simulink model "Wrapper_oClientServer_Model"  (R2024b)
settings: Solver=FixedStepDiscrete  StartTime=0.0  StopTime=10.0  FixedStep=0.05  RelTol=1e-3
undefined symbols (not defined in the file or in its folder): call_ServerService_getDataC, call_ServerService_setDataA, call_ServerService_setDataB, DataA, DataB, sut_ServerService_setDataA, sut_ServerService_setDataB, sut_step
settings Model: Tag=EP_AA_WRAPPER_TOPLEVEL  DataDictionary=Wrapper_oClientServer_Model.sldd  Creator=nabilekhoury  LastModifiedBy=nabilekhoury
settings OptimizationCC: DefaultParameterBehavior=Inlined  OptimizeBlockIOStorage=off  BufferReuse=off  ReuseModelBlockBuffer=off  GlobalBufferReuse=off  ExpressionFolding=off  EnableMemcpy=off  PassReuseOutputArgsAs=Individual arguments  LocalBlockOutputs=off  ZeroExternalMemoryAtStartup=off  ZeroInternalMemoryAtStartup=off  OptimizeDataStoreBuffers=off  BusAssignmentInplaceUpdate=off  OptimizationLevel=level0  OptimizationCustomize=off  EfficientTunableParamExpr=on
settings DebuggingCC: ParameterTunabilityLossMsg=error
settings ModelReferenceCC: ModelReferenceNumInstancesAllowed=Single
settings SFSimCC: MATLABDynamicMemAlloc=off  SimTargetLang=C++
settings RTWCC: Description=Embedded Coder  SystemTargetFile=ert.tlc  GenCodeOnly=on  TemplateMakefile=ert_default_tmf  CustomSourceCode="#include \"oClientServer_Model_adapter.h\""  CustomInitializer=sut_initialize();  TargetLang=C++
settings CodeAppCC: ForceParamTrailComments=on  IgnoreCustomStorageClasses=off  MaxIdLength=256  OperatorAnnotations=on  SimulinkDataObjDesc=on  SFDataObjDesc=on  CustomSymbolStrGlobalVar=w_$R$N$M  CustomSymbolStrType=w_$N$R$M_T  InsertBlockDesc=on
settings ERTTargetCC: TargetLangStandard=C++17 (ISO)  GenerateSampleERTMain=on  SupportAbsoluteTime=off  SupportNonFinite=off  SupportComplex=off  RootIOFormat=Structure reference  ERTCustomFileTemplate=example_file_process.tlc

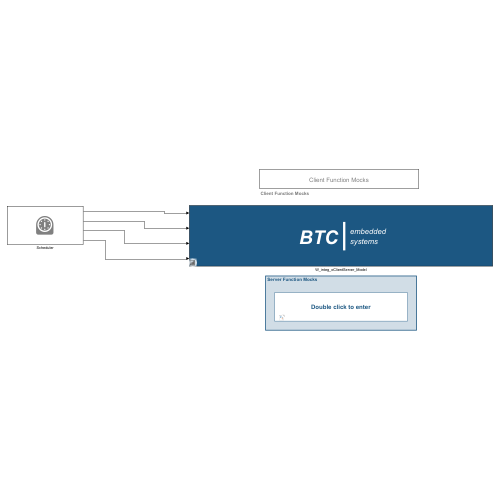
[thumbnail: Simulink's stored preview of the top-level diagram]
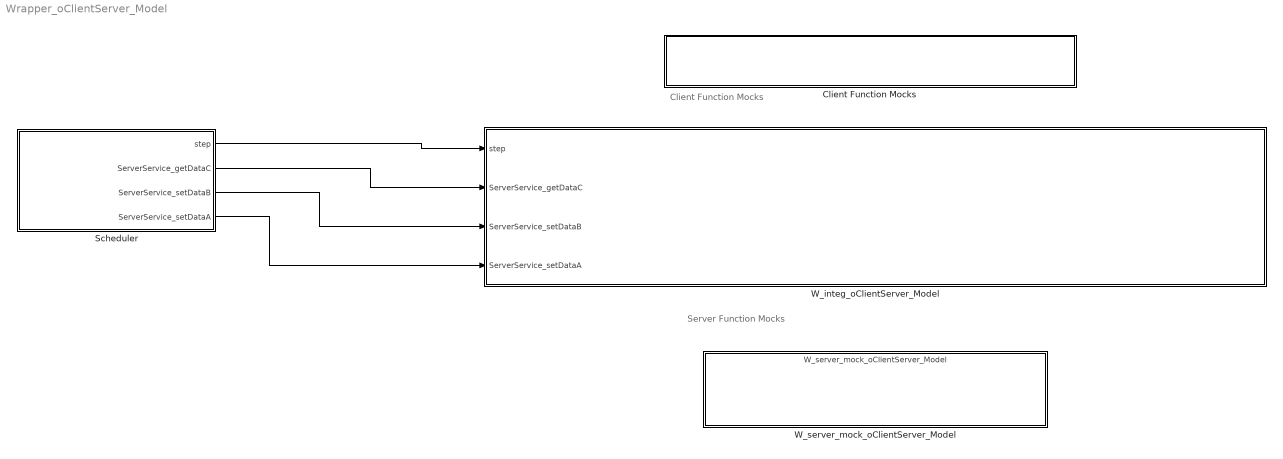
== system Wrapper_oClientServer_Model ==
  note: Client Function Mocks
  note: Server Function Mocks
  Client Function Mocks : Subsystem
      mask Display: color('gray'); disp('{\fontsize{16}Client Function Mocks}', 'texmode', 'on');
  Scheduler : Subsystem
      mask Display: disp('\color{gray}\fontsize{50}⏲', 'texmode', 'on');
  W_integ_oClientServer_Model : Subsystem  Variant=on  VariantControlMode=label  LabelModeActiveChoice=orig  PropagateVariantConditions=on
      settings: OpenFcn=open_system(gcb, 'mask');
      mask DialogControl DescGroupVar Prompt: BTC Embedded Systems SUT block
      mask DialogControl DescTextVar Prompt: This is the BTC Embedded Systems SUT block, referencing the original Adaptive AUTOSAR model.
      mask DialogControl DescButVar Prompt: Open original model...
      mask DialogControl DescButVar Callback: open_system('oClientServer_Model');
      mask Display: disp('\color{white}\it\fontsize{20}                          embedded\newline                          systems', 'texmode', 'on');disp('{{\color{white}\bf\fontsize{50}\it   BTC}  \fontsize{80}|      \color{black}\fontsize{20}\newline }', 'texmode','on');
  W_server_mock_oClientServer_Model : ModelReference  ModelNameDialog=W_server_mock_oClientServer_Model  SimulationMode=Normal  ScheduleRates=on  ModelReferenceVersion=1.1
      mask Display: disp('{\bf\fontsize{16}Double click to enter}', 'texmode', 'on');
  wires:
  Scheduler/2(ServerService_getDataC) -> W_integ_oClientServer_Model/2(ServerService_getDataC)
  Scheduler/4(ServerService_setDataA) -> W_integ_oClientServer_Model/4(ServerService_setDataA)
  Scheduler/3(ServerService_setDataB) -> W_integ_oClientServer_Model/3(ServerService_setDataB)
  Scheduler/1(step) -> W_integ_oClientServer_Model/1(step)

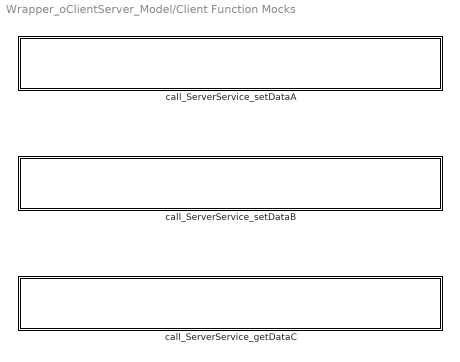
== system Wrapper_oClientServer_Model/Client Function Mocks ==
  call_ServerService_getDataC : Subsystem  TreatAsAtomicUnit=on
  call_ServerService_setDataA : Subsystem  TreatAsAtomicUnit=on
  call_ServerService_setDataB : Subsystem  TreatAsAtomicUnit=on

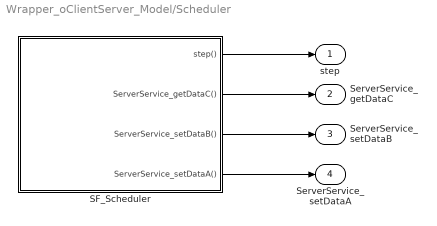
== system Wrapper_oClientServer_Model/Scheduler ==
  SF_Scheduler : Stateflow chart  TreatAsAtomicUnit=on
  step : Outport
  ServerService_getDataC : Outport  Port=2
  ServerService_setDataB : Outport  Port=3
  ServerService_setDataA : Outport  Port=4
  wires:
  SF_Scheduler/1(step()) -> step/1
  SF_Scheduler/2(ServerService_getDataC()) -> ServerService_getDataC/1
  SF_Scheduler/3(ServerService_setDataB()) -> ServerService_setDataB/1
  SF_Scheduler/4(ServerService_setDataA()) -> ServerService_setDataA/1

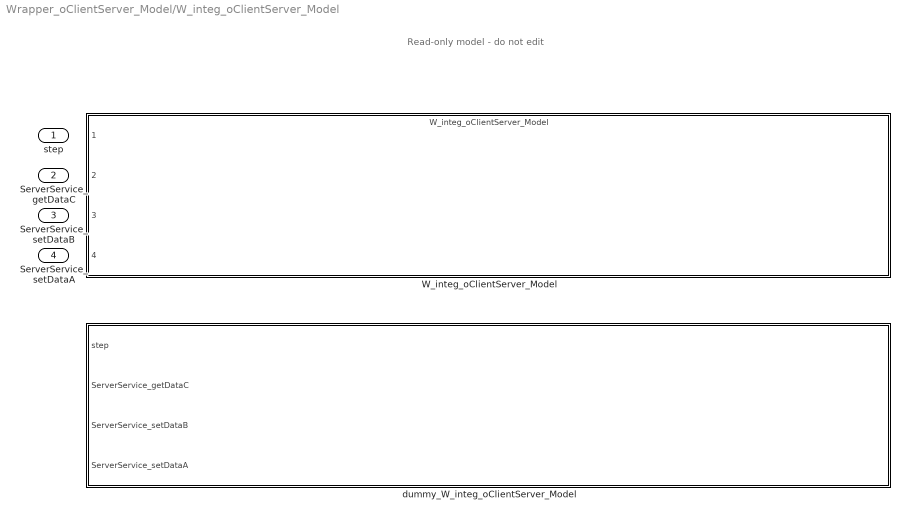
== system Wrapper_oClientServer_Model/W_integ_oClientServer_Model ==
  note: Read-only model - do not edit
  step : Inport
  ServerService_getDataC : Inport  Port=2
  ServerService_setDataB : Inport  Port=3
  ServerService_setDataA : Inport  Port=4
  W_integ_oClientServer_Model : ModelReference  Tag=BTC AUTOSAR Main Model Reference Block  ModelNameDialog=W_integ_oClientServer_Model  SimulationMode=Normal  ScheduleRates=on  VariantControl=orig  ModelReferenceVersion=1.2
  dummy_W_integ_oClientServer_Model : Subsystem  VariantControl=dummy

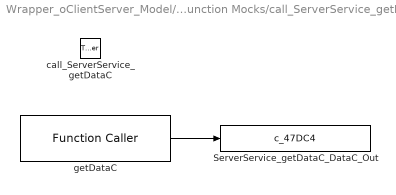
== system Wrapper_oClientServer_Model/Client Function Mocks/call_ServerService_getDataC ==
  call_ServerService_getDataC : TriggerPort  TriggerType=function-call  IsSimulinkFunction=on  FunctionName=call_ServerService_getDataC  VariantControl=(inherit)
  ServerService_getDataC_DataC_Out : DataStoreWrite  DataStoreName=c_47DC4  IndexOptions=Index vector (dialog)  Indices=1  OutputSizes=1
  getDataC : FunctionCaller  FunctionPrototype=DataC = sut_ServerService_getDataC()  OutputArgumentSpecifications=double(0)
  wires:
  getDataC/1 -> ServerService_getDataC_DataC_Out/1

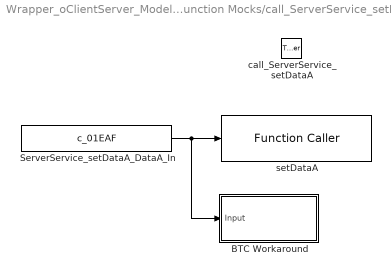
== system Wrapper_oClientServer_Model/Client Function Mocks/call_ServerService_setDataA ==
  call_ServerService_setDataA : TriggerPort  TriggerType=function-call  IsSimulinkFunction=on  FunctionName=call_ServerService_setDataA  VariantControl=(inherit)
  BTC Workaround : Subsystem
      settings: OpenFcn=open_system(gcb, 'mask');
      mask DialogControl DescGroupVar Prompt: BTC Embedded Systems MIL stabilizer
      mask DialogControl DescTextVar Prompt: The BTC Embedded Systems MIL stabilizer prevents a known Matlab 2023b issue that results in a crash. It has no effect on the signal. Do not edit its contents.
      mask Display: disp('\color[rgb]{0.11,0.34,0.51}\bf MIL stabilizer', 'texmode', 'on');
  ServerService_setDataA_DataA_In : DataStoreRead  DataStoreName=c_01EAF  IndexOptions=Index vector (dialog)  Indices=1  OutputSizes=1
  setDataA : FunctionCaller  FunctionPrototype=sut_ServerService_setDataA(DataA)  InputArgumentSpecifications=double(0)
  wires:
  ServerService_setDataA_DataA_In/1 -> setDataA/1, BTC Workaround/1(Input)

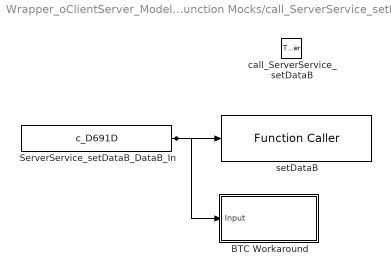
== system Wrapper_oClientServer_Model/Client Function Mocks/call_ServerService_setDataB ==
  call_ServerService_setDataB : TriggerPort  TriggerType=function-call  IsSimulinkFunction=on  FunctionName=call_ServerService_setDataB  VariantControl=(inherit)
  BTC Workaround : Subsystem
      settings: OpenFcn=open_system(gcb, 'mask');
      mask DialogControl DescGroupVar Prompt: BTC Embedded Systems MIL stabilizer
      mask DialogControl DescTextVar Prompt: The BTC Embedded Systems MIL stabilizer prevents a known Matlab 2023b issue that results in a crash. It has no effect on the signal. Do not edit its contents.
      mask Display: disp('\color[rgb]{0.11,0.34,0.51}\bf MIL stabilizer', 'texmode', 'on');
  ServerService_setDataB_DataB_In : DataStoreRead  DataStoreName=c_D691D  IndexOptions=Index vector (dialog)  Indices=1  OutputSizes=1
  setDataB : FunctionCaller  FunctionPrototype=sut_ServerService_setDataB(DataB)  InputArgumentSpecifications=double(0)
  wires:
  ServerService_setDataB_DataB_In/1 -> setDataB/1, BTC Workaround/1(Input)

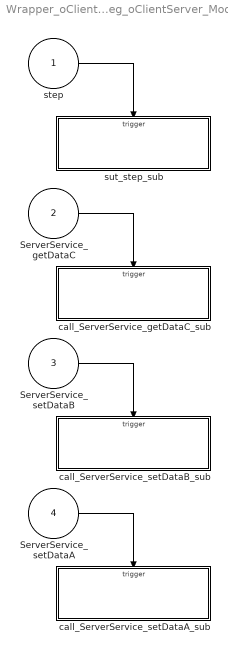
== system Wrapper_oClientServer_Model/W_integ_oClientServer_Model/dummy_W_integ_oClientServer_Model ==
  step : Inport  OutputFunctionCall=on
  ServerService_getDataC : Inport  Port=2  OutputFunctionCall=on
  ServerService_setDataB : Inport  Port=3  OutputFunctionCall=on
  ServerService_setDataA : Inport  Port=4  OutputFunctionCall=on
  call_ServerService_getDataC_sub : Subsystem  TreatAsAtomicUnit=on
  call_ServerService_setDataA_sub : Subsystem  TreatAsAtomicUnit=on
  call_ServerService_setDataB_sub : Subsystem  TreatAsAtomicUnit=on
  sut_step_sub : Subsystem  TreatAsAtomicUnit=on
  wires:
  step/1 -> sut_step_sub/Trigger
  ServerService_getDataC/1 -> call_ServerService_getDataC_sub/Trigger
  ServerService_setDataB/1 -> call_ServerService_setDataB_sub/Trigger
  ServerService_setDataA/1 -> call_ServerService_setDataA_sub/Trigger

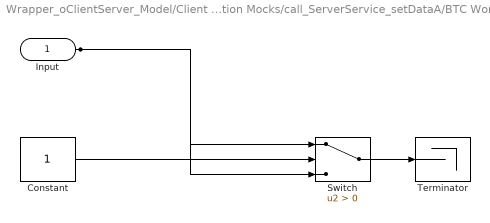
== system Wrapper_oClientServer_Model/Client Function Mocks/call_ServerService_setDataA/BTC Workaround ==
  Input : Inport
  Constant : Constant
  Switch : Switch  Criteria=u2 > Threshold  SaturateOnIntegerOverflow=off  InputSameDT=off
  Terminator : Terminator
  wires:
  Input/1 -> Switch/1, Switch/3
  Switch/1 -> Terminator/1
  Constant/1 -> Switch/2

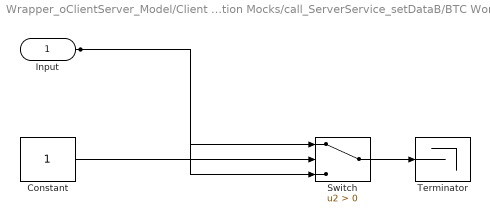
== system Wrapper_oClientServer_Model/Client Function Mocks/call_ServerService_setDataB/BTC Workaround ==
  Input : Inport
  Constant : Constant
  Switch : Switch  Criteria=u2 > Threshold  SaturateOnIntegerOverflow=off  InputSameDT=off
  Terminator : Terminator
  wires:
  Input/1 -> Switch/1, Switch/3
  Switch/1 -> Terminator/1
  Constant/1 -> Switch/2

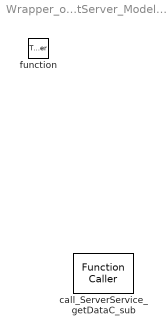
== system Wrapper_oClientServer_Model/W_integ_oClientServer_Model/dummy_W_integ_oClientServer_Model/call_ServerService_getDataC_sub ==
  function : TriggerPort  TriggerType=function-call  VariantControl=(inherit)
  call_ServerService_getDataC_sub : FunctionCaller  FunctionPrototype=call_ServerService_getDataC()  InputArgumentSpecifications=<Enter example>  OutputArgumentSpecifications=<Enter example>

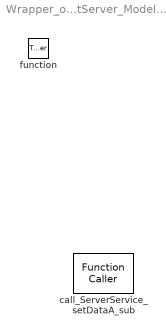
== system Wrapper_oClientServer_Model/W_integ_oClientServer_Model/dummy_W_integ_oClientServer_Model/call_ServerService_setDataA_sub ==
  function : TriggerPort  TriggerType=function-call  VariantControl=(inherit)
  call_ServerService_setDataA_sub : FunctionCaller  FunctionPrototype=call_ServerService_setDataA()  InputArgumentSpecifications=<Enter example>  OutputArgumentSpecifications=<Enter example>

== system Wrapper_oClientServer_Model/W_integ_oClientServer_Model/dummy_W_integ_oClientServer_Model/call_ServerService_setDataB_sub ==
  function : TriggerPort  TriggerType=function-call  VariantControl=(inherit)
  call_ServerService_setDataB_sub : FunctionCaller  FunctionPrototype=call_ServerService_setDataB()  InputArgumentSpecifications=<Enter example>  OutputArgumentSpecifications=<Enter example>

== system Wrapper_oClientServer_Model/W_integ_oClientServer_Model/dummy_W_integ_oClientServer_Model/sut_step_sub ==
  function : TriggerPort  TriggerType=function-call  VariantControl=(inherit)
  sut_step_sub : FunctionCaller  FunctionPrototype=sut_step()  InputArgumentSpecifications=<Enter example>  OutputArgumentSpecifications=<Enter example>

== stateflow chart Wrapper_oClientServer_Model/Scheduler/SF_Scheduler ==
  state Schedule
    en:
    send(step);
    send(ServerService_getDataC);
    send(ServerService_setDataB);
    send(ServerService_setDataA);
    du:
    on every(1, tick):send(step);
    on every(1, tick):send(ServerService_getDataC);
    on every(1, tick):send(ServerService_setDataB);
    on every(1, tick):send(ServerService_setDataA);
  (default) -> Schedule : /*Update the Order/Rate/Asynchronous calls of the runnables*/
  events: step output FUNCTION_CALL_EVENT; ServerService_getDataC output FUNCTION_CALL_EVENT; ServerService_setDataB output FUNCTION_CALL_EVENT; ServerService_setDataA output FUNCTION_CALL_EVENT
